simulink model "SimpleShaft_Working"  (R2023b)
settings: Solver=ode1  StartTime=0.0  StopTime=25  FixedStep=.4  RelTol=1e-3
values from neighbouring files (symbols this model uses):
  A = 4    [Week1_WorkingCode.m]
  B = [10,0.1]    [Project_1.m]    (also in Week1_WorkingCode.m = 1)
  J = 1    [Week1_WorkingCode.m]
  w_0 = W_0(z)    [Project_1.m]    (also in Week1_WorkingCode.m = 1)
settings Model: Creator=nakro  LastModifiedBy=nakro

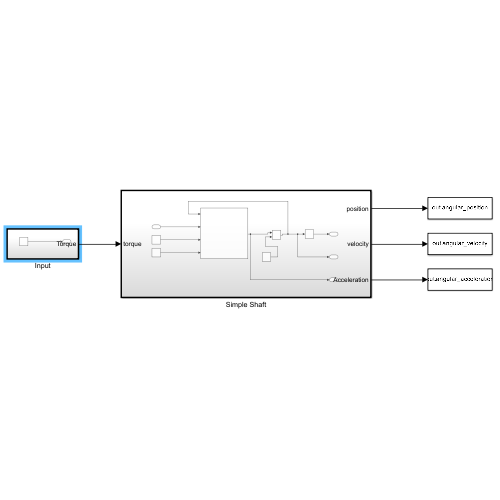
[thumbnail: Simulink's stored preview of the top-level diagram]
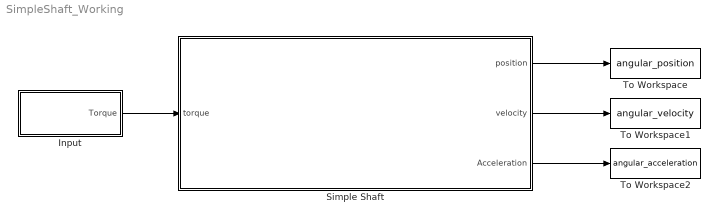
== system SimpleShaft_Working ==
  Input : Subsystem  TreatAsAtomicUnit=on
  Simple Shaft : Subsystem  TreatAsAtomicUnit=on
  To Workspace : ToWorkspace  VariableName=angular_position  SaveFormat=Timeseries  SampleTime=-1
  To Workspace1 : ToWorkspace  VariableName=angular_velocity  SaveFormat=Timeseries  SampleTime=-1
  To Workspace2 : ToWorkspace  VariableName=angular_acceleration  SaveFormat=Timeseries  SampleTime=-1
  wires:
  Simple Shaft/1(position) -> To Workspace/1
  Simple Shaft/2(velocity) -> To Workspace1/1
  Input/1(Torque) -> Simple Shaft/1(torque)
  Simple Shaft/3(Acceleration) -> To Workspace2/1

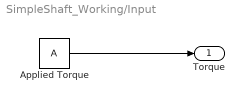
== system SimpleShaft_Working/Input ==
  Applied Torque : Constant  Value=A
  Torque : Outport
  wires:
  Applied Torque/1 -> Torque/1

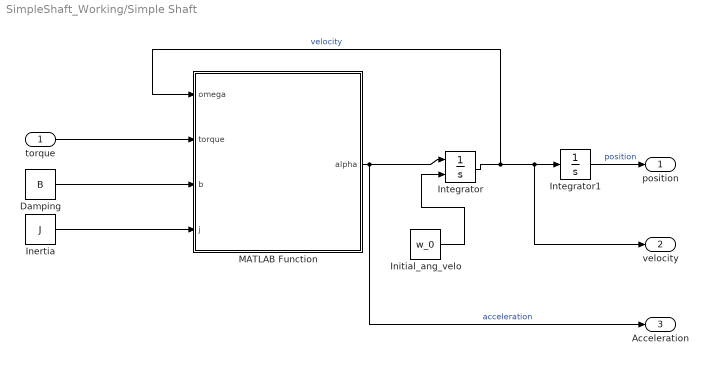
== system SimpleShaft_Working/Simple Shaft ==
  torque : Inport
  Damping : Constant  Value=B
  Inertia : Constant  Value=J
  Initial_ang_velo : Constant  Value=w_0
  Integrator : Integrator  InitialConditionSource=external  InitialCondition=w_0
  Integrator1 : Integrator
  MATLAB Function : MATLAB Function  TreatAsAtomicUnit=on
  position : Outport
  velocity : Outport  Port=2
  Acceleration : Outport  Port=3
  wires:
  MATLAB Function/1(alpha) -> Integrator/1, Acceleration/1  "acceleration"
  Integrator/1 -> MATLAB Function/1(omega), velocity/1, Integrator1/1  "velocity"
  Damping/1 -> MATLAB Function/3(b)
  Inertia/1 -> MATLAB Function/4(j)
  Integrator1/1 -> position/1  "position"
  torque/1 -> MATLAB Function/2(torque)
  Initial_ang_velo/1 -> Integrator/2

== matlab function SimpleShaft_Working/Simple Shaft/MATLAB Function ==
  data: omega input; alpha output; torque input; b input; j input
function alpha = fcn(omega,torque,b,j) 

alpha = (torque - omega *b)/j;

end
